simulink model "Ecat_Test_Example"  (R2016a)
settings: Solver=FixedStepDiscrete  StartTime=0.0  StopTime=60  FixedStep=1/1000  RelTol=1e-3
libraries: SOEM_EtherCAT_Lib x5
settings Model: SimulationMode=external  Creator=RecSet  LastModifiedBy=root
settings DataIOCC: LimitDataPoints=on  SaveFormat=Array
settings DebuggingCC: SolverPrmCheckMsg=warning  AllowSymbolicDim=off
settings HardwareCC: ProdBitPerLong=64  ProdLongLongMode=on  ProdHWDeviceType=Intel->x86-64 (Linux 64)
settings ModelReferenceCC: PropagateSignalLabelsOutOfModel=off
settings RTWCC: Description=Generic Real-Time Target  CustomInclude=/usr/local/include/soem  CustomLibrary=/usr/local/lib/libsoem.so  Toolchain=GNU gcc/g++ v4.4.x | gmake (64-bit Linux)  BuildConfiguration=Faster Runs
settings CodeAppCC: MaxIdLength=95
settings GRTTargetCC: TargetLangStandard=C99 (ISO)  ExtMode=on
settings ConfigComp: CovModelRefEnable=Off  CovSFcnEnable=off

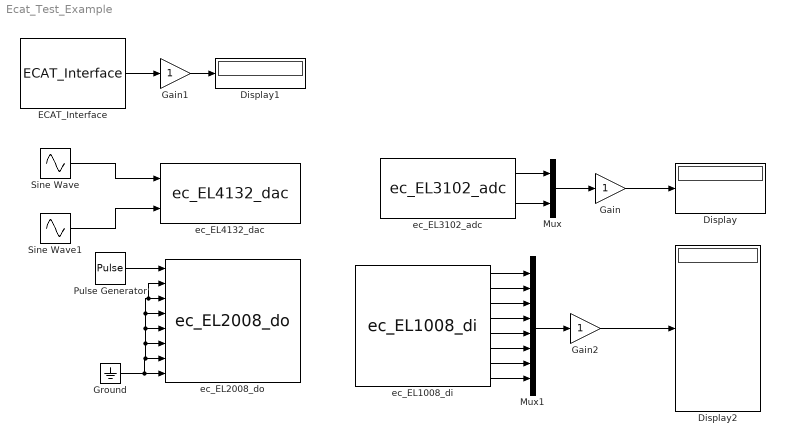
== system Ecat_Test_Example ==
  Display : Display
  Display1 : Display
  Display2 : Display
  ECAT_Interface : SOEM_EtherCAT_Lib/ECAT_Interface  Priority=0  IFINTERFACE=eth0  TS=1/1000
  Gain : Gain
  Gain1 : Gain  OutDataTypeStr=double
  Gain2 : Gain
  Ground : Ground
  Mux : Mux  Inputs=2
  Mux1 : Mux  Inputs=8
  Pulse Generator : DiscretePulseGenerator  PulseType=Time based  Period=.5  PulseWidth=50
  Sine Wave : Sin  Amplitude=10  Frequency=2*pi*.2  SampleTime=0
  Sine Wave1 : Sin  Amplitude=10  Frequency=2*pi*.2  Phase=pi  SampleTime=0
  ec_EL1008_di : SOEM_EtherCAT_Lib/ec_EL1008_di  LINKID=1
  ec_EL2008_do : SOEM_EtherCAT_Lib/ec_EL2008_do  LINKID=1
  ec_EL3102_adc : SOEM_EtherCAT_Lib/ec_EL3102_adc  LINKID=1
  ec_EL4132_dac : SOEM_EtherCAT_Lib/ec_EL4132_dac  LINKID=1
  wires:
  Gain/1 -> Display/1
  ECAT_Interface/1 -> Gain1/1
  Gain1/1 -> Display1/1
  Mux1/1 -> Gain2/1
  Gain2/1 -> Display2/1
  Sine Wave/1 -> ec_EL4132_dac/1
  Sine Wave1/1 -> ec_EL4132_dac/2
  Pulse Generator/1 -> ec_EL2008_do/1
  Ground/1 -> ec_EL2008_do/2, ec_EL2008_do/3, ec_EL2008_do/4, ec_EL2008_do/5, ec_EL2008_do/6, ec_EL2008_do/7, ec_EL2008_do/8
  ec_EL3102_adc/1 -> Mux/1
  ec_EL3102_adc/2 -> Mux/2
  Mux/1 -> Gain/1
  ec_EL1008_di/7 -> Mux1/7
  ec_EL1008_di/5 -> Mux1/5
  ec_EL1008_di/1 -> Mux1/1
  ec_EL1008_di/4 -> Mux1/4
  ec_EL1008_di/8 -> Mux1/8
  ec_EL1008_di/2 -> Mux1/2
  ec_EL1008_di/6 -> Mux1/6
  ec_EL1008_di/3 -> Mux1/3
